simulink model "Tankvol_check"  (R2023a)
settings: Solver=FixedStepAuto  StartTime=0.0  StopTime=0.  FixedStep=1.0  RelTol=1e-3
settings Model: Creator=horty  LastModifiedBy=horty
settings DataIOCC: SignalLogging=off  DSMLogging=off  SaveTime=off  ReturnWorkspaceOutputs=off

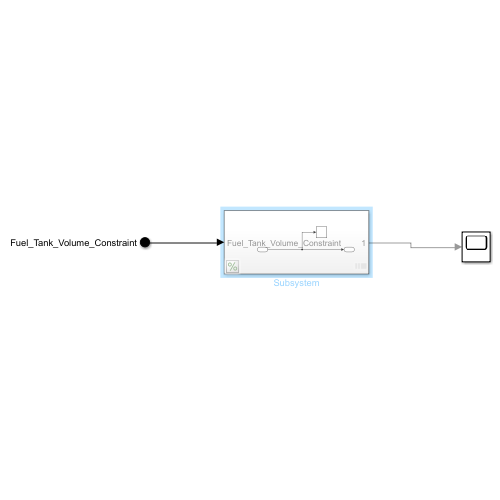
[thumbnail: Simulink's stored preview of the top-level diagram]
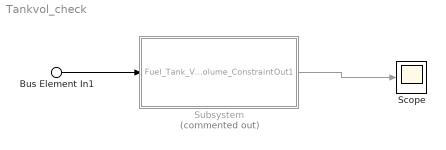
== system Tankvol_check ==
  Bus Element In1 : Inport  PortName=Fuel_Tank_Volume_Constraint
  Scope : Scope
  Subsystem : Subsystem  Commented=on
  wires:
  Bus Element In1/1 -> Subsystem/1(Fuel_Tank_Volume_Constraint)
  Subsystem/1(Out1) -> Scope/1

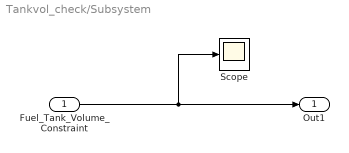
== system Tankvol_check/Subsystem ==
  Fuel_Tank_Volume_Constraint : Inport
  Scope : Scope
  Out1 : Outport
  wires:
  Fuel_Tank_Volume_Constraint/1 -> Scope/1, Out1/1
